simulink model "adaptor1"  (R2014b)
settings: Solver=ode45  StartTime=0.0  StopTime=10.0  RelTol=1e-3
settings Model: Creator=ravoson  LastModifiedBy=ravoson

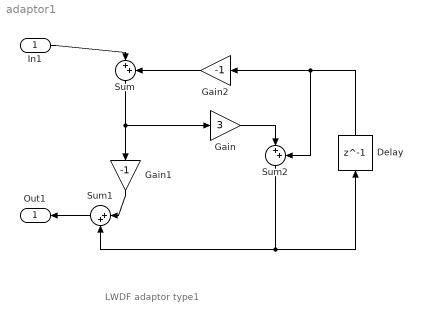
== system adaptor1 ==
  note: LWDF adaptor type1
  In1 : Inport
  Delay : Delay  DelayLength=1  InitialCondition=0
  Gain : Gain  Gain=3
  Gain1 : Gain  Gain=-1
  Gain2 : Gain  Gain=-1
  Sum : Sum  Inputs=|++
      settings: AttributesFormatString=%<Tag>
  Sum1 : Sum  Inputs=|++
  Sum2 : Sum  Inputs=|++
  Out1 : Outport
  wires:
  Sum/1 -> Gain/1, Gain1/1
  Gain2/1 -> Sum/2
  In1/1 -> Sum/1
  Gain/1 -> Sum2/1
  Delay/1 -> Sum2/2, Gain2/1
  Gain1/1 -> Sum1/1
  Sum2/1 -> Sum1/2, Delay/1
  Sum1/1 -> Out1/1
